simulink model "v21pid"  (R2021a)
settings: Solver=VariableStepAuto  StartTime=0.0  StopTime=inf  RelTol=1e-3
undefined symbols (not defined in the file): PLC1
libraries: opclib x6, simulink_extras x4, pid_lib x1
settings Model: Creator=123  LastModifiedBy=adb

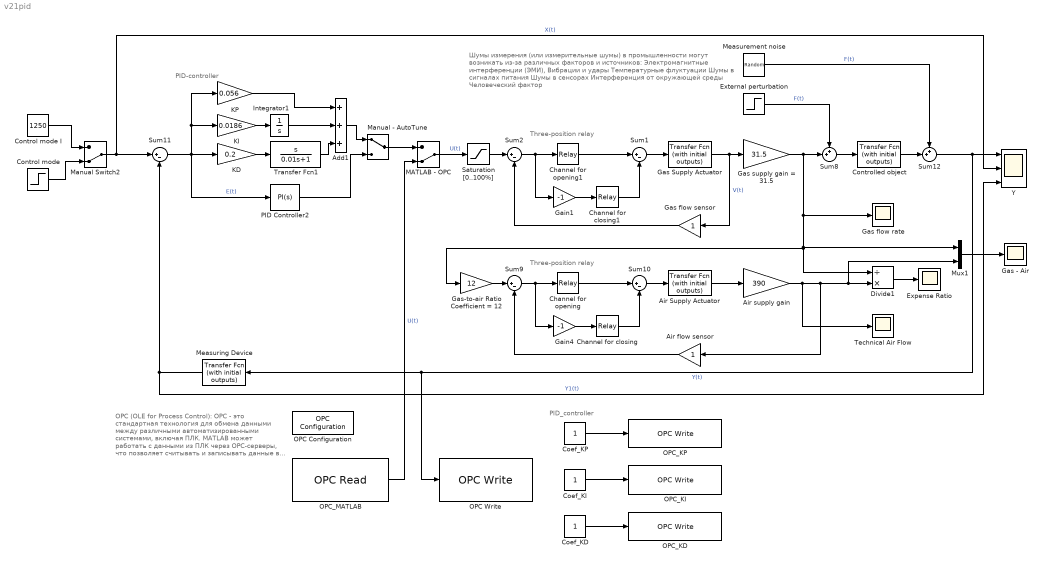
== system v21pid ==
  note: Шумы измерения (или измерительные шумы) в промышленности могут возникать из-за различных факторов и источников:
      | Электромагнитные интерференции (ЭМИ),
      | Вибрации и удары
      | Температурные флуктуации
      | Шумы в сигналах питания
      | Шумы в сенсорах
      | Интерференция от окружающей среды
      | Человеческий фактор
  note: OPC (OLE for Process Control): OPC - это стандартная технология для обмена данными между различными автоматизированными системами, включая ПЛК. MATLAB может работать с данными из ПЛК через OPC-серверы, что позволяет считывать и записывать данные в переменные ПЛК.
  note: PID_controller
  note: PID-controller
  note: Three-position relay
  note: Three-position relay
  Add1 : Sum  Inputs=+++
  Air Supply Actuator : simulink_extras/Additional Linear/Transfer Fcn (with initial outputs)  N=[100]  D="[1.2  0]"  Y0=69.93  U0=0
  Air flow sensor : Gain
  Air supply gain : Gain  Gain=390
  Channel for opening : Relay  OnSwitchValue=20  OffSwitchValue=0
  Channel for opening1 : Relay  OnSwitchValue=0.1  OffSwitchValue=0
  Channel for closing : Relay  OnSwitchValue=20  OffSwitchValue=0
  Channel for closing1 : Relay  OnSwitchValue=0.1  OffSwitchValue=0
  Coef_KD : Constant
  Coef_KI : Constant
  Coef_KP : Constant
  Control mode : Step  Time=10  Before=800  After=1300  SampleTime=0
  Control mode I : Constant  Value=1250
  Controlled object : simulink_extras/Additional Linear/Transfer Fcn (with initial outputs)  N=0.528  D=[12 1]  Y0=800  U0=800/0.528
  Divide1 : Product  Inputs=/*
  Expense Ratio : Scope
  External perturbation : Step  Time=100  After=-500  SampleTime=0
  Gain1 : Gain  Gain=-1
  Gain4 : Gain  Gain=-1
  Gas - Air : Scope
  Gas Supply Actuator : simulink_extras/Additional Linear/Transfer Fcn (with initial outputs)  N=[100]  D="[1.2  0]"  Y0=48.1  U0=0
  Gas flow rate : Scope
  Gas flow sensor : Gain
  Gas supply gain = 31.5 : Gain  Gain=31.5
  Gas-to-air Ratio Coefficient = 12 : Gain  Gain=12
  Integrator1 : Integrator  InitialCondition=48.1
  KD : Gain  Gain=0.2
  KI : Gain  Gain=0.0186
  KP : Gain  Gain=0.056
  MATLAB - OPC : ManualSwitch  CurrentSetting=0
  Manual - AutoTune : ManualSwitch
  Manual Switch2 : ManualSwitch  CurrentSetting=0
  Measurement noise : UniformRandomNumber  Minimum=-0.015  Maximum=0.015  SampleTime=0.1
  Measuring Device : simulink_extras/Additional Linear/Transfer Fcn (with initial outputs)  N=[1]  D="[0.48  1]"  Y0=800  U0=800
  Mux1 : Mux  Inputs=2
  OPC Configuration : opclib/OPC Configuration  opcServers=localhost/CoDeSys.OPC.02/100  errMissingItems=Error  errReadWrite=Warn  errShutdown=Error  errRTViolation=Warn  rtEnable=on  speedup=1  showLatency=off  beingUsed=on
      settings: SourceProductBaseCode=OT
  OPC Write : opclib/OPC Write  serverHost=localhost  serverID=CoDeSys.OPC.02  itemIDs=PLC1:.act_temp  writeMode=Synchronous  updateRate=0.1
      settings: SourceProductBaseCode=OT
  OPC_KD : opclib/OPC Write  serverHost=localhost  serverID=CoDeSys.OPC.02  itemIDs=PLC1:.KD  writeMode=Synchronous  updateRate=0.1
      settings: SourceProductBaseCode=OT
  OPC_KI : opclib/OPC Write  serverHost=localhost  serverID=CoDeSys.OPC.02  itemIDs=PLC1:.KI  writeMode=Synchronous  updateRate=0.1
      settings: SourceProductBaseCode=OT
  OPC_KP : opclib/OPC Write  serverHost=localhost  serverID=CoDeSys.OPC.02  itemIDs=PLC1:.KP  writeMode=Synchronous  updateRate=0.1
      settings: SourceProductBaseCode=OT
  OPC_MATLAB : opclib/OPC Read  serverHost=localhost  serverID=CoDeSys.OPC.02  itemIDs=PLC1:.Temp_out  readMode=Synchronous (cache)  dataType=double  updateRate=0.1  showQual=off  showTS=off  tsMode=Seconds since start
      settings: SourceProductBaseCode=OT
  PID Controller2 : pid_lib/PID Controller  Controller=PI  Form=Parallel  TimeDomain=Continuous-time  UseExternalTs=off  SampleTime=-1  IntegratorMethod=Forward Euler  FilterMethod=Forward Euler  ControllerParametersSource=internal  P=0.43  I=0.043  D=0.34  UseFilter=on  N=100  TunerSelectOption=Transfer Function Based (PID Tuner App)  InitialConditionSource=internal  InitialConditionForIntegrator=48.1  InitialConditionForFilter=0  DifferentiatorICPrevScaledInput=0  ExternalReset=none  TrackingMode=off  Kt=1  LimitOutput=off  SatLimitsSource=internal  UpperSaturationLimit=inf  LowerSaturationLimit=-inf  LinearizeAsGain=on  AntiWindupMode=none  Kb=1  POutMin=[]  POutMax=[]  IOutMin=[]  IOutMax=[]  DOutMin=[]  DOutMax=[]  NOutMin=[]  NOutMax=[]  SumOutMin=[]  SumOutMax=[]  SaturationOutMin=[]  SaturationOutMax=[]  PParamMin=[]  PParamMax=[]  IParamMin=[]  IParamMax=[]  DParamMin=[]  DParamMax=[]  NParamMin=[]  NParamMax=[]  KbParamMin=[]  KbParamMax=[]  KtParamMin=[]  KtParamMax=[]  KbOutMin=[]  KbOutMax=[]  KtOutMin=[]  KtOutMax=[]  IntegratorOutMin=[]  IntegratorOutMax=[]  FilterOutMin=[]  FilterOutMax=[]  SumI1OutMin=[]  SumI1OutMax=[]  SumI2OutMin=[]  SumI2OutMax=[]  SumI3OutMin=[]  SumI3OutMax=[]  SumI4OutMin=[]  SumI4OutMax=[]  SumDOutMin=[]  SumDOutMax=[]  DifferentiatorOutMin=[]  DifferentiatorOutMax=[]  FilterDiffOutCoefMin=[]  FilterDiffOutCoefMax=[]  ReciprocalOutMin=[]  ReciprocalOutMax=[]  SumDenOutMin=[]  SumDenOutMax=[]  SumNumOutMin=[]  SumNumOutMax=[]  DivideOutMin=[]  DivideOutMax=[]  UdiffTsProdOutMin=[]  UdiffTsProdOutMax=[]  NTsProdOutMin=[]  NTsProdOutMax=[]  UintegralTsProdOutMin=[]  UintegralTsProdOutMax=[]  UngainTsProdOutMin=[]  UngainTsProdOutMax=[]  IntegratorContinuousStateAttributes=''  IntegratorStateMustResolveToSignalObject=off  IntegratorRTWStateStorageClass=Auto  FilterContinuousStateAttributes=''  FilterStateMustResolveToSignalObject=off  FilterRTWStateStorageClass=Auto  ParallelPVariant=InternalParameters  IdealPVariant=Disabled  IVariant=InternalParameters  DVariant=Disabled  IntegratorVariant=Continuous  SatVariant=Disabled  AWVariant=Passthrough  PCopyVariant=Disabled  TRVariant=Disabled  FdbkBlocksVariant=Forward  IdealPFdbkVariant=Disabled  SatFdbkVariant=Disabled  DerivativeFilterVariant=Disabled  NVariant=Disabled  NCopyVariant=Disabled_SignalSpec  FilterICVariant=Disabled  IntegratorICVariant=InternalICs  ExternalResetVariant=Disabled  TRSumVariant=Passthrough  SumFdbkVariant=Disabled  SumVariant=Sum_PI  TsampFilterVariant=InternalTs  TsampNgainVariant=Passthrough  TsampIntegralVariant=Passthrough  ExternalSaturationOutDataTypeStr=Inherit: Same as second input
  Saturation [0..100%] : Saturate  UpperLimit=100  LowerLimit=0
  Sum{1..2,9..11} (5 alike) : Sum  Inputs=|+-
  Sum12 : Sum  Inputs=++|
  Sum8 : Sum  Inputs=++|
  Technical Air Flow : Scope
  Transfer Fcn1 : TransferFcn  Numerator=[1 0]  Denominator=[0.01 1]
  Y : Scope  NumInputPorts=3
  wires:
  PID Controller2/1 -> Manual - AutoTune/2
  Gas Supply Actuator/1 -> Gas supply gain = 31.5/1, Gas flow sensor/1  "V(t)"
  External perturbation/1 -> Sum8/1  "F(t)"
  Add1/1 -> Manual - AutoTune/1
  Gas supply gain = 31.5/1 -> Sum8/2, Gas flow rate/1, Gas-to-air Ratio Coefficient = 12/1, Divide1/1, Mux1/1
  Sum9/1 -> Channel for opening/1, Gain4/1
  Channel for opening/1 -> Sum10/1
  KP/1 -> Add1/1
  Saturation [0..100%]/1 -> Sum2/1
  Mux1/1 -> Gas - Air/1
  Gas flow sensor/1 -> Sum2/2
  KI/1 -> Integrator1/1
  KD/1 -> Transfer Fcn1/1
  Measurement noise/1 -> Sum12/1  "F(t)"
  Air supply gain/1 -> Technical Air Flow/1, Air flow sensor/1, Mux1/2, Divide1/2
  Controlled object/1 -> Sum12/2
  Sum10/1 -> Air Supply Actuator/1
  Divide1/1 -> Expense Ratio/1
  Channel for closing/1 -> Sum10/2
  Air Supply Actuator/1 -> Air supply gain/1
  Gain4/1 -> Channel for closing/1
  Gas-to-air Ratio Coefficient = 12/1 -> Sum9/1
  Sum8/1 -> Controlled object/1
  Measuring Device/1 -> Sum11/2, Y/3  "Y1(t)"
  Control mode I/1 -> Manual Switch2/1
  MATLAB - OPC/1 -> Saturation [0..100%]/1  "U(t)"
  Manual - AutoTune/1 -> MATLAB - OPC/1
  Sum11/1 -> PID Controller2/1, KD/1, KP/1, KI/1  "E(t)"
  Sum12/1 -> Y/1, OPC Write/1, Measuring Device/1  "Y(t)"
  Manual Switch2/1 -> Sum11/1, Y/2  "X(t)"
  Control mode/1 -> Manual Switch2/2
  Integrator1/1 -> Add1/2
  Sum2/1 -> Channel for opening1/1, Gain1/1
  Channel for opening1/1 -> Sum1/1
  Channel for closing1/1 -> Sum1/2
  Gain1/1 -> Channel for closing1/1
  Sum1/1 -> Gas Supply Actuator/1
  Air flow sensor/1 -> Sum9/2
  Coef_KP/1 -> OPC_KP/1
  Coef_KI/1 -> OPC_KI/1
  Coef_KD/1 -> OPC_KD/1
  OPC_MATLAB/1 -> MATLAB - OPC/2  "U(t)"
  Transfer Fcn1/1 -> Add1/3
